simulink model "AUV_Nonlinear_Dynamic_Model"  (R2019b)
settings: Solver=VariableStepAuto  StartTime=0.0  StopTime=10.0  RelTol=1e-3
settings Model: Creator=7385281  LastModifiedBy=7385281

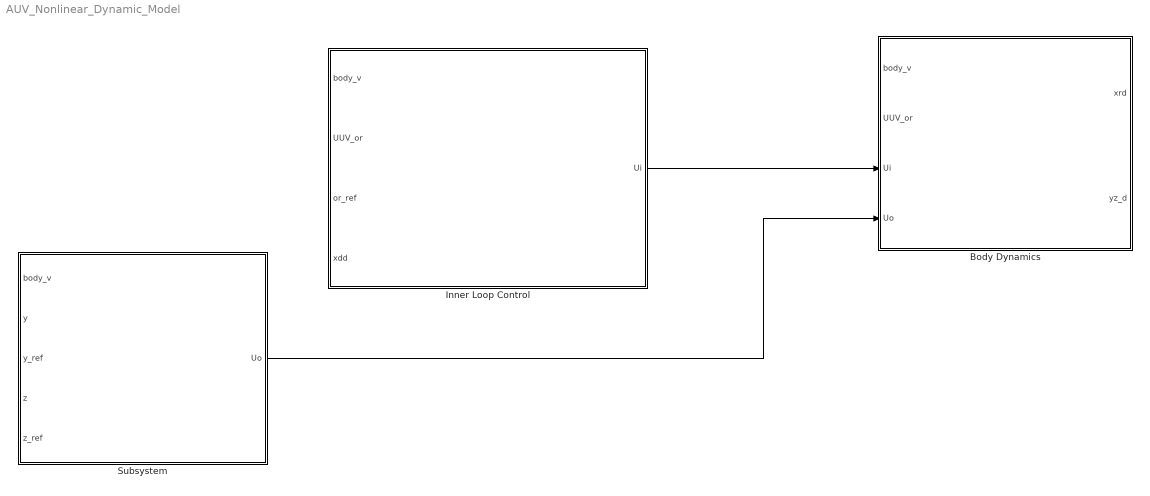
== system AUV_Nonlinear_Dynamic_Model ==
  Body Dynamics : Subsystem
  Inner Loop Control : Subsystem
  Subsystem : Subsystem
  wires:
  Inner Loop Control/1(Ui) -> Body Dynamics/3(Ui)
  Subsystem/1(Uo) -> Body Dynamics/4(Uo)

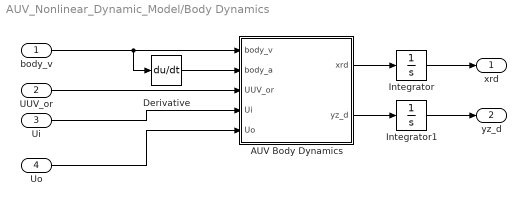
== system AUV_Nonlinear_Dynamic_Model/Body Dynamics ==
  body_v : Inport
  UUV_or : Inport  Port=2
  Ui : Inport  Port=3
  Uo : Inport  Port=4
  AUV Body Dynamics : MATLAB Function  TreatAsAtomicUnit=on
  Derivative : Derivative
  Integrator : Integrator
  Integrator1 : Integrator
  xrd : Outport
  yz_d : Outport  Port=2
  wires:
  AUV Body Dynamics/1(xrd) -> Integrator/1
  Integrator/1 -> xrd/1
  AUV Body Dynamics/2(yz_d) -> Integrator1/1
  Integrator1/1 -> yz_d/1
  body_v/1 -> Derivative/1, AUV Body Dynamics/1(body_v)
  Derivative/1 -> AUV Body Dynamics/2(body_a)
  UUV_or/1 -> AUV Body Dynamics/3(UUV_or)
  Ui/1 -> AUV Body Dynamics/4(Ui)
  Uo/1 -> AUV Body Dynamics/5(Uo)

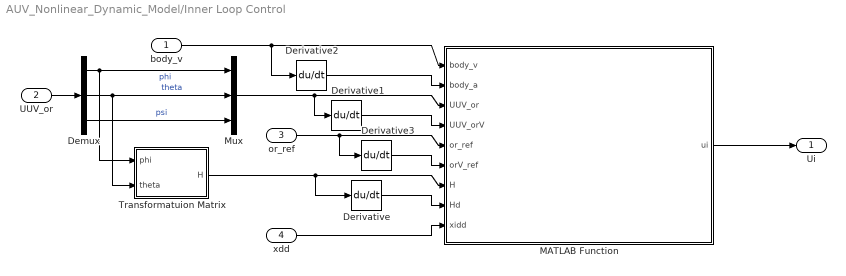
== system AUV_Nonlinear_Dynamic_Model/Inner Loop Control ==
  body_v : Inport
  UUV_or : Inport  Port=2
  or_ref : Inport  Port=3
  xdd : Inport  Port=4
  Demux : Demux  Outputs=3
  Derivative{,1..3} (4 alike) : Derivative
  MATLAB Function : MATLAB Function  TreatAsAtomicUnit=on
  Mux : Mux  Inputs=3
  Transformatuion Matrix : MATLAB Function  TreatAsAtomicUnit=on
  Ui : Outport
  wires:
  body_v/1 -> Derivative2/1, MATLAB Function/1(body_v)
  Demux/1 -> Mux/1, Transformatuion Matrix/1(phi)  "phi"
  Mux/1 -> Derivative1/1, MATLAB Function/3(UUV_or)
  Derivative/1 -> MATLAB Function/8(Hd)
  Derivative1/1 -> MATLAB Function/4(UUV_orV)
  UUV_or/1 -> Demux/1
  Derivative2/1 -> MATLAB Function/2(body_a)
  MATLAB Function/1(ui) -> Ui/1
  Demux/2 -> Mux/2, Transformatuion Matrix/2(theta)  "theta"
  or_ref/1 -> Derivative3/1, MATLAB Function/5(or_ref)
  Derivative3/1 -> MATLAB Function/6(orV_ref)
  Transformatuion Matrix/1(H) -> Derivative/1, MATLAB Function/7(H)
  xdd/1 -> MATLAB Function/9(xidd)
  Demux/3 -> Mux/3  "psi"

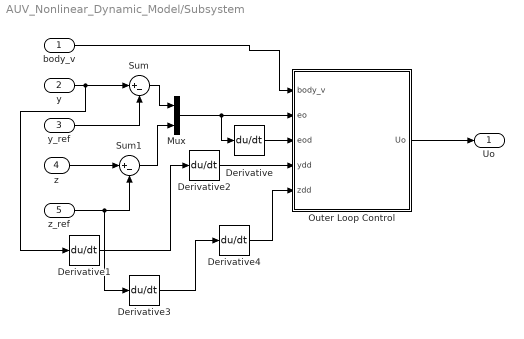
== system AUV_Nonlinear_Dynamic_Model/Subsystem ==
  body_v : Inport
  y : Inport  Port=2
  y_ref : Inport  Port=3
  "z " : Inport  Port=4
  z_ref : Inport  Port=5
  Derivative{,1..4} (5 alike) : Derivative
  Mux : Mux  Inputs=2
  Outer Loop Control : MATLAB Function  TreatAsAtomicUnit=on
  Sum : Sum  Inputs=|+-
  Sum1 : Sum  Inputs=|+-
  Uo : Outport
  wires:
  body_v/1 -> Outer Loop Control/1(body_v)
  y/1 -> Derivative1/1, Sum/1
  y_ref/1 -> Sum/2
  z_ref/1 -> Sum1/2, Derivative3/1
  "z "/1 -> Sum1/1
  Sum/1 -> Mux/1
  Sum1/1 -> Mux/2
  Mux/1 -> Derivative/1, Outer Loop Control/2(eo)
  Derivative/1 -> Outer Loop Control/3(eod)
  Derivative2/1 -> Outer Loop Control/4(ydd)
  Derivative1/1 -> Derivative2/1
  Derivative4/1 -> Outer Loop Control/5(zdd)
  Derivative3/1 -> Derivative4/1
  Outer Loop Control/1(Uo) -> Uo/1

== matlab function AUV_Nonlinear_Dynamic_Model/Inner Loop Control/Transformatuion Matrix ==
  data: phi input; H output; theta input
function H = fcn(phi,theta)
% This function takes in two orientation angles of the AUV and caluclates
% the transformation matrix H
%%%%%%%%%%%%%%%%%%%%%%%%%%%%%%%%%%%%%%%%%%%%%%%%%%%%%%%%%%%%%%%%%%%%%%%%%%%
% INPUTS:
    % phi -roll angle, about x axis
    % theta - pitch angle, about y axis
% OUTPUTS: 
    % H - 2x2 transormation matrix
%%%%%%%%%%%%%%%%%%%%%%%%%%%%%%%%%%%%%%%%%%%%%%%%%%%%%%%%%%%%%%%%%%%%%%%%%%%
% Main Code:
% Calculate transformation matrix

H = [cos(phi) -sin(phi); sin(phi)/cos(theta) cos(phi)/cos(theta)];

== matlab function AUV_Nonlinear_Dynamic_Model/Inner Loop Control/MATLAB Function ==
  data: body_v input; ui output; body_a input; UUV_or input; UUV_orV input; or_ref input; orV_ref input; H input; Hd input; xidd input
function ui =inner_loop_control(body_v,body_a, UUV_or, UUV_orV, or_ref, orV_ref, H,Hd,xidd)
% Ben Colvin
% The purpose of this function is to calculate the inner loop control
% vector for the control of the UUV
%%%%%%%%%%%%%%%%%%%%%%%%%%%%%%%%%%%%%%%%%%%%%%%%%%%%%%%%%%%%%%%%%%%%%%%%%%%
% INPUTS:
    % body_v - 6x1 vector of body fixed velocities:
        % u - surge velocity
        % v - sway velocity
        % w - heading velocity
        % p - roll velocity
        % q - pitch velocity
        % r - yaw velocity
    % body_a - 6x1 vector of body fixed accelerations
        % ud - surge acceleration
        % vd - sway acceleration
        % wd - heading acceleration
        % pd - roll acceleration
        % qd - pitch acceleration
        % rd - yaw acceleration
    % World fixed terms:
    % UUV_or - 2x1 vector orientation of UUV, theta, psi
        % theta - current orientation of UUV
        % psi - current orientation of UUV
    
    % UUV_orV - 2x1 vector of angular velocity thetad, psid
        % thetad - current orientation velocity of UUV
        % psid - current orentation velocity of UUV
    % or_ref -2x1 vector refernce orientation theta, psi
        % theta_ref - refernce orientation of UUV
        % psi_ref - reference orientation of UUV
    % orV_ref - 2x1 vector reference angular veloities thetad,psid
        % theta_refd - reference orientation velocity of UUV
        % psi_refd - refernce orientation velocity of UUV
    % H - 2x2 transformation matrix
    % Hd - 2x2 derivative of transformation matrix
    % xr - body rates state vector [q r]'
        
% OUTPUTS:
    % ui - control output of inner loop, to be used in the AUV dynamics

% CONSTANTS
    a1 = 1; % control constant (not set) * must be +
    a2 = 1; % control constant (not set) * must be +
    k1 = 1; % control constant (not set)
    k2 = 1; % control constant (not set)
% GLOBAL PARAMETERS:
    global m
    global Ix
    global Iy
    global Iz
    global Tp
    global Mwd
    global Mrp
    global Mq
    global Mqd
    global Mw
    global MwwQ
    global MqqQ
    global Nrd
    global Nvd
    global Npq
    global Nr
    global Nv
    global NrrQ
    global NvvQ
    global xg
    global xb
    global yg
    global yb
    global zg
    global zb
    global W
    global B
%%%%%%%%%%%%%%%%%%%%%%%%%%%%%%%%%%%%%%%%%%%%%%%%%%%%%%%%%%%%%%%%%%%%%%%%%%%
% INPUT INITIALIZATION:

% Body Fixed Velocity initialization
u = body_v(1);
v = body_v(2);
w = body_v(3);
p = body_v(4);
q = body_v(5);
r = body_v(6);
xr = [q r]';

% Body fixed acceleration initialization
ud = body_a(1);
vd = body_a(2);
wd = body_a(3);
pd = body_a(4);
qd = body_a(5);
rd = body_a(6);
        
% UUV orientation
phi = UUV_or(1)
theta = UUV_or(2);
psi = UUV_or(3);

% UUV angular velocities
phid = UUV_orV(1);
thetad = UUV_orV(2);
psid = UUV_orV(3);

% UUV orientation reference
theta_ref = or_ref(1);
psi_ref = or_ref(2);

%UUV angular velocity reference
theta_refd = orV_ref(1);
psi_refd = orV_ref(2);
%%%%%%%%%%%%%%%%%%%%%%%%%%%%%%%%%%%%%%%%%%%%%%%%%%%%%%%%%%%%%%%%%%%%%%%%%%%

% Main Code:

% Ar, Br is the differential equation system of the body rate dynamics
% xrd = Ar + Br*u, where u is the input to the DE
Ar = [-(((Ix-Iz)*r*p+m*(zg*(ud-v*r+w*q)-xg*(wd-u*q+v*p)))+Mqd*qd+Mwd*wd+Mrp*r*p+Mq*u*q)/(Iy-Mqd)+(Mw*u*w+MwwQ*w*abs(w)+MqqQ*q*abs(q)-(xg*W-xb*B)*cos(theta)*cos(phi)-(zg*W-zb*B)*sin(theta))/(Iy-Mqd);...
    -(((Iy-Ix)*p*q+m*(xg*(vd-w*p+u*r)-yg*(ud-v*r+w*q)))+Nrd*rd+Nvd*vd+Npq*p*q+Nr*u*r)/(Iz-Nrd)+(Nv*u*v+NrrQ*r*abs(r)+NvvQ*v*abs(v)-(xg*W-xb*B)*cos(theta)*sin(phi)+(yg*W-yb*B)*sin(theta))/(Iz-Nrd)];

`


% inner states error vector
ei = [theta - theta_ref; psi - psi_ref];

% inner state velocity error vector
eid = [thetad - theta_refd; psid - psi_refd];

% null control constants (not set)
k = [k1; k2];

% Positive Constant matrix (not set)
D = [a1 0; 0 a2];




% Controls Coeffecient Row Vector funtion A_i(x_i,t)
Ai = 2*ei' * D * H *Br;

% Controls Load Scalar Function
Bi = [-2*ei'*D*(-xidd+Hd+H*(x^-1)); xi+H*Ar-2*eid'*D*eid; -2*c1*ei'*D*eid-c2*eid];

% MPGI of Ai
Ai_plus = Ai'/(Ai*Ai');

% null projection matrix
Pi = eye(2) - Ai_plus*Ai;

% null control vector
lamda = k*eid';

% Control output 2x1 matrix delta_theta, delta_psi 
ui = Ai_plus*Bi+Pi*lamda;

== matlab function AUV_Nonlinear_Dynamic_Model/Body Dynamics/AUV Body Dynamics ==
  data: body_v input; xrd output; body_a input; UUV_or input; Ui input; Uo input; yz_d output
function [xrd,yz_d] = fcn(body_v,body_a, UUV_or,Ui,Uo)
%%%%%%%%%%%%%%%%%%%%%%%%%%%%%%%%%%%%%%%%%%%%%%%%%%%%%%%%%%%%%%%%%%%%%%%%%%%
% INPUTS:
% body_v - 6x1 vector of body fixed velocities:
        % u - surge velocity
        % v - sway velocity
        % w - heading velocity
        % p - roll velocity
        % q - pitch velocity
        % r - yaw velocity
    % body_a - 6x1 vector of body fixed accelerations
        % ud - surge acceleration
        % vd - sway acceleration
        % wd - heading acceleration
        % pd - roll acceleration
        % qd - pitch acceleration
        % rd - yaw acceleration
    % World fixed terms:
    % UUV_or - 2x1 vector orientation of UUV, theta, psi
        % theta - current orientation of UUV
        % psi - current orientation of UUV
     % Ui - inner loop input control vector [delta_theta; delta_psi]
     % Uo - outer loop input control vector [tri_y; tri_z]
% OUTPUTS:
    % xrd - body rate dynamics derivative [q_dot r_dot]' 
% CONSTANTS:
% GLOBAL PARAMETERS:
    global m
    global Ix
    global Iy
    global Iz
    global Tp
    global Mwd
    global Mrp
    global Mq
    global Mqd
    global Mw
    global MwwQ
    global MqqQ
    global Nrd
    global Nvd
    global Npq
    global Nr
    global Nv
    global NrrQ
    global NvvQ
    global xg
    global xb
    global yg
    global yb
    global zg
    global zb
    global W
    global B
%%%%%%%%%%%%%%%%%%%%%%%%%%%%%%%%%%%%%%%%%%%%%%%%%%%%%%%%%%%%%%%%%%%%%%%%%%%
% INPUT INITIALIZATION

% Body Fixed Velocity initialization
u = body_v(1);
v = body_v(2);
w = body_v(3);
p = body_v(4);
q = body_v(5);
r = body_v(6);
xr = [q r]';

% Body fixed acceleration initialization
ud = body_a(1);
vd = body_a(2);
wd = body_a(3);
pd = body_a(4);
qd = body_a(5);
rd = body_a(6);
        
% UUV orientation
phi = UUV_or(1)
theta = UUV_or(2);
psi = UUV_or(3);
xr = [theta; psi];

%%%%%%%%%%%%%%%%%%%%%%%%%%%%%%%%%%%%%%%%%%%%%%%%%%%%%%%%%%%%%%%%%%%%%%%%%%%
% MAIN CODE:

% ATTITUDE DYNAMICS
% Ar, Br is the differential equation system of the body rate dynamics

Ar = [-(((Ix-Iz)*r*p+m*(zg*(ud-v*r+w*q)-xg*(wd-u*q+v*p)))+Mqd*qd+Mwd*wd+Mrp*r*p+Mq*u*q)/(Iy-Mqd)+(Mw*u*w+MwwQ*w*abs(w)+MqqQ*q*abs(q)-(xg*W-xb*B)*cos(theta)*cos(phi)-(zg*W-zb*B)*sin(theta))/(Iy-Mqd);...
    -(((Iy-Ix)*p*q+m*(xg*(vd-w*p+u*r)-yg*(ud-v*r+w*q)))+Nrd*rd+Nvd*vd+Npq*p*q+Nr*u*r)/(Iz-Nrd)+(Nv*u*v+NrrQ*r*abs(r)+NvvQ*v*abs(v)-(xg*W-xb*B)*cos(theta)*sin(phi)+(yg*W-yb*B)*sin(theta))/(Iz-Nrd)];

Br = [0 -Tp*xr/(Iy-Mqd) 0; 0 0 Tp*xr/(Iz-Nrd)];

% Differential Equation of Body rate dynamics
xrd = Ar + Br*Ui;

% POSITION DYNAMICS
% M matrix terms
M11 = -u*sin(theta)*sin(psi)+v*sin(phi)*cos(theta)*sin(psi)+w*cos(phi)*cos(theta)*sin(psi);
M12 = u*cos(theta)*cos(psi)+v*(sin(phi)*sin(theta)*cos(psi)-cos(phi)*sin(psi))+w*(sin(phi)*sin(psi)-cos(phi)*sin(theta)*cos(phi));
M21 = -u*cos(theta) - v*sin(theta)*sin(phi)-w*sin(theta)*cos(phi);
M22 = 0;

% N matrix terms
N11 = u*cos(theta)*sin(psi) + v*(sin(phi)*sin(theta)*sin(psi)+cos(phi)*cos(psi))+w*(sin(theta)*cos(psi)*sin(psi)-sin(phi)*cos(psi));
N21 = -u*sin(theta) + v*sin(phi)*cos(theta) + w*cos(psi)*cos(theta);

M = [M11 M12; M21 M22];
N = [N11; N21];

% dereivative of position vector of outer loop control
yz_d = M*Uo + N;

== matlab function AUV_Nonlinear_Dynamic_Model/Subsystem/Outer Loop Control ==
  data: body_v input; eo input; eod input; Uo output; ydd input; zdd input
function Uo =outer_loop_control(body_v,eo, eod,ydd,zdd)
% Ben Colvin
% The purpose of this function is to calculate the inner loop control
% vector for the control of the UUV
%%%%%%%%%%%%%%%%%%%%%%%%%%%%%%%%%%%%%%%%%%%%%%%%%%%%%%%%%%%%%%%%%%%%%%%%%%%
% INPUTS:
    % body_v - 6x1 vector of body fixed velocities:
        % u - surge velocity
        % v - sway velocity
        % w - heading velocity
        % p - roll velocity
        % q - pitch velocity
        % r - yaw velocity
    % eo - 2x1 state error vector [y_e; z_e]
    % eod - 2x1 velocity error vector [yd_e; zd_e]
    % ydd - acceleration in y direction of global system
    % zdd - acceleration in z direction of global system
    
% OUTPUTS:
    % Uo - control output of outer loop, to be used in the AUV dynamics

% CONSTANTS
    a1 = 1; % control constant (not set) * must be +
    a2 = 1; % control constant (not set) * must be +
    a3 = 1; % control constant (not set)
    a4 = 1; % control constant (not set)
    k1 = 1; % control constant (not set)
    k2 = 1; % control constant (not set)
% GLOBAL PARAMETERS:
    global L
    global dia
    global m
    global Ix
    global Iy
    global Iz
    global Tp
    global Mwd
    global Mrp
    global Mq
    global Mqd
    global Mw
    global MwwQ
    global MqqQ
    global Nrd
    global Nvd
    global Npq
    global Nr
    global Nv
    global NrrQ
    global NvvQ
    global xg
    global xb
    global yg
    global yb
    global zg
    global zb
    global W
    global B
%%%%%%%%%%%%%%%%%%%%%%%%%%%%%%%%%%%%%%%%%%%%%%%%%%%%%%%%%%%%%%%%%%%%%%%%%%%
% INPUT INITIALIZATION:

% Body Fixed Velocity initialization
u = body_v(1);
v = body_v(2);
w = body_v(3);
p = body_v(4);
q = body_v(5);
r = body_v(6);

% Outer Position Acceleration Vector
xo_dd = [ydd; zdd];

% Control Constants
D12 = [a1 0; 0 a2];
D34 = [a3 0; 0 a4];
k_o = [k1; k2];

%%%%%%%%%%%%%%%%%%%%%%%%%%%%%%%%%%%%%%%%%%%%%%%%%%%%%%%%%%%%%%%%%%%%%%%%%%%
% MAIN CODE:

% M matrix terms
M11 = -u*sin(theta)*sin(psi)+v*sin(phi)*cos(theta)*sin(psi)+w*cos(phi)*cos(theta)*sin(psi);
M12 = u*cos(theta)*cos(psi)+v*(sin(phi)*sin(theta)*cos(psi)-cos(phi)*sin(psi))+w*(sin(phi)*sin(psi)-cos(phi)*sin(theta)*cos(phi));
M21 = -u*cos(theta) - v*sin(theta)*sin(phi)-w*sin(theta)*cos(phi);
M22 = 0;

N11 = u*cos(theta)*sin(psi) + v*(sin(phi)*sin(theta)*sin(psi)+cos(phi)*cos(psi))+w*(sin(theta)*cos(psi)*sin(psi)-sin(phi)*cos(psi));
N21 = -u*sin(theta) + v*sin(phi)*cos(theta) + w*cos(psi)*cos(theta);

M = [M11 M12; M21 M22];
N = [N11; N21];



% Dynamics
Ao = 2*eo'*D34*M;
Bo = 2*eo'*D12*(xo_dd-N)+2*eod'*D12*eod+2*c1*eo'*D12*eod+c2*eo'*D12*eo;

% Adjunct Matrix A*
Ao_star = adjoint(Ao);

% Moore-Penrose Generealized Inverse
Ao_plus = (Ao_star*Ao)^-1 * Ao_star;

% Null Projection Matrix for outer loop
Po = eye(2) - Ao_plus*Ao;

% Null Control Vector
lamda_o = k_o*eod';

% Outer Loop Control Input [triangle_psi; triagnle _theta]
Uo = Ao_plus*Bo+Po*lamda_o;
